simulink model "final_sim"  (R2024b)
settings: Solver=FixedStepAuto  StartTime=0.0  StopTime=10  FixedStep=step_size  RelTol=1e-3
values from neighbouring files (symbols this model uses):
  F_alphas = zeros([4,8])    [make_polynomial.m]
  Ic = I    (= 0)    [quadcopter_tmp_par.m]
  m = 4    [inertia.m]    (also in quadcopter_tmp_par.m)
  M_RB = [ m*eye(3) , zeros(3) ; zeros(3) , Ic2 ]    [inertia.m]    (also in quadcopter_tmp_par.m = [m*eye(3),zeros(3);zeros(3),Ic])
libraries: vrlib x3, aerolibutil x2, sharedtransform x2, simulink_extras x1, sharedutil x1
settings Model: Creator=vince  LastModifiedBy=vince

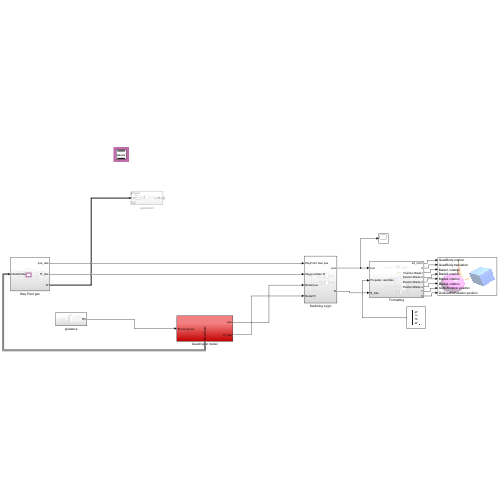
[thumbnail: Simulink's stored preview of the top-level diagram]
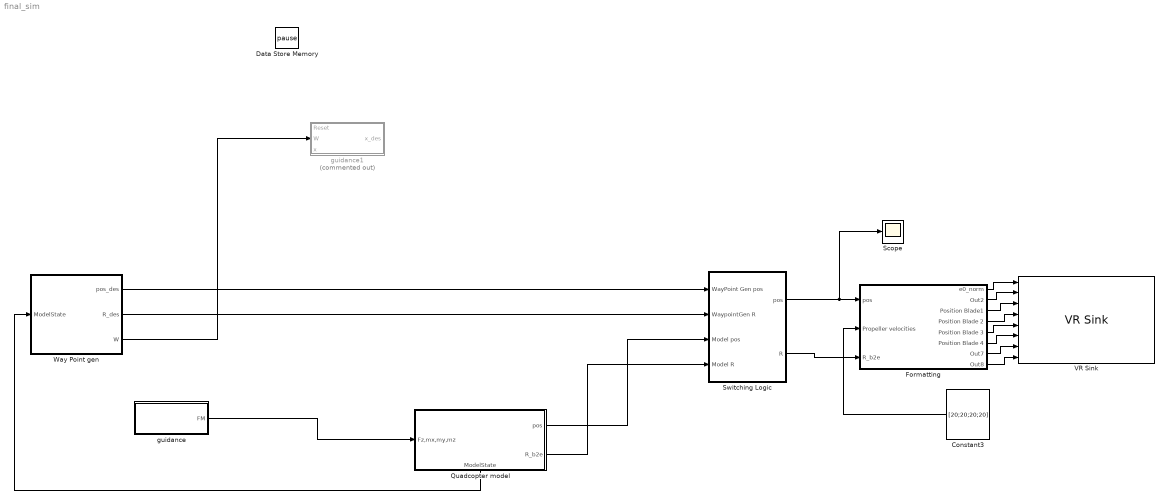
== system final_sim ==
  Constant3 : Constant  Value=[20;20;20;20]  VectorParams1D=off
  Data Store Memory : DataStoreMemory  DataStoreName=pause  WriteAfterWriteMsg=warning  ShowAdditionalParam=off  OutDataTypeStr=boolean
  Formatting : Subsystem
  Quadcopter model : Subsystem
      settings: PortSchema="{\"entries\":[{\"content\":{\"sides\":[{\"content\":{\"connectorIds\":[\"In1\"]},\"type\":\"ConnectorPlacement.EquallySpacedRectSide\",\"uuid\":\"b95d4d67-ceb1-468a-a740-70bed9055261\"},{\"content\":{\"connectorIds\":[\"Out1\",\"Out2\"],\"side\":\"RIGHT\"},\"type\":\"ConnectorPlacement.EquallySpacedRectSide\",\"uuid\":\"d9e2e888-327b-4c74-9853-42e66e59dabe\"},{\"content\":{\"side\":\"TOP\"},\"type\":\"ConnectorPlacement.EquallySpacedRectSide\",\"uuid\":\"f1e6c0a4-a009-4e38-aaef-f99bc46a780f\"},{\"content\":{\"connectorIds\":[\"Out3\"],\"side\":\"BOTTOM\"},\"type\":\"ConnectorPlacement.EquallySpacedRectSide\",\"uuid\":\"26785e0d-8be3-430d-abc1-8d415326c7f3\"}]},\"type\":\"ConnectorPlacement.EquallySpacedConnector\",\"uuid\":\"bfffa9f4-9135-40ac-b83a-608bfe18c3a4\"}],\"packageUris\":[\"http://schema.mathworks.com/mf0/Connector/R2020b\"],\"version\":\"1.0\"}"
  Scope : Scope
  Switching Logic : Subsystem
  VR Sink : vrlib/VR Sink  InstantiateOnLoad=on  SampleTime=12*0.005  ViewEnable=on  RemoteChange=off  RemoteView=off  FieldsWritten=QuadBody.rotation.4.1.1.double#QuadBody.translation.3.1.1.double#Blade1.rotation.4.1.1.double#Blade3.rotation.4.1.1.double#Blade2.rotation.4.1.1.double#Blade4.rotation.4.1.1.double#IsoNoRotation.position.3.1.1.double#OnQuadNoRotation.position.3.1.1.double  WorldFileName=Quadcopter_VR.wrl  AutoView=on  VideoDimensions=[]  AllowVariableSize=off  FigureProperties="{'Position', 'Name', 'Viewpoint', 'CameraBound', 'CameraDirection', 'CameraPosition', 'CameraUpVector', 'ZoomFactor', 'Antialiasing', 'Headlight', 'Lighting', 'Sound', 'StatusBar', 'Stereo3D', 'Stereo3DCameraOffset', 'Stereo3DHIT', 'ToolBar', 'Textures', 'Transparency', 'Triad', 'Wireframe', 'NavZones', 'NavMode', 'NavSpeed', 'CaptureFileFormat', 'CaptureFileName', 'Record2DCompressMethod', 'Record2DCompressQuality', 'Record2D', 'Record2DFileName', 'Record2DFPS', 'NavPanel'; [1.9301428571428571e+03   6.0471428571428555e+02   5.7600000000000000e+02   3.5000000000000000e+02], '', 'Chase - No Rotation', 'on', [0.0000000000000000e+00   0.0000000000000000e+00  -1.0000000000000000e+00], [0.0000000000000000e+00   0.0000000000000000e+00   0.0000000000000000e+00], [0.0000000000000000e+00   1.0000000000000000e+00   0.0000000000000000e+00], [1.0000000000000000e+00], 'on', 'on', 'on', 'on', 'on', 'off', [1.0000000149011612e-01], [0.0000000000000000e+00], 'on', 'on', 'on', 'none', 'off', 'off', 'fly', 'normal', 'tif', '%f_anim_%n.tif', 'auto', [7.5000000000000000e+01], 'off', '%f_anim_%n.avi', 'auto', 'halfbar'}"
  Way Point gen : Subsystem
  guidance : Subsystem
  guidance1 : Subsystem  Commented=on
  wires:
  Formatting/6(Position Blade 4) -> VR Sink/6
  Formatting/8(Out8) -> VR Sink/8
  Formatting/1(e0_norm) -> VR Sink/1
  Switching Logic/2(R) -> Formatting/3(R_b2e)
  Formatting/4(Position Blade 2) -> VR Sink/4
  Formatting/3(Position Blade1) -> VR Sink/3
  Formatting/7(Out7) -> VR Sink/7
  Formatting/5(Position Blade 3) -> VR Sink/5
  guidance/1(FM) -> Quadcopter model/1(Fz,mx,my,mz)
  Formatting/2(Out2) -> VR Sink/2
  Constant3/1 -> Formatting/2(Propeller velocities)
  Switching Logic/1(pos) -> Scope/1, Formatting/1(pos)
  Way Point gen/2(R_des) -> Switching Logic/2(WaypointGen R)
  Way Point gen/3(W) -> guidance1/2(W)
  Quadcopter model/2(R_b2e) -> Switching Logic/4(Model R)
  Way Point gen/1(pos_des) -> Switching Logic/1(WayPoint Gen pos)
  Quadcopter model/1(pos) -> Switching Logic/3(Model pos)
  Quadcopter model/3(ModelState) -> Way Point gen/1(ModelState)

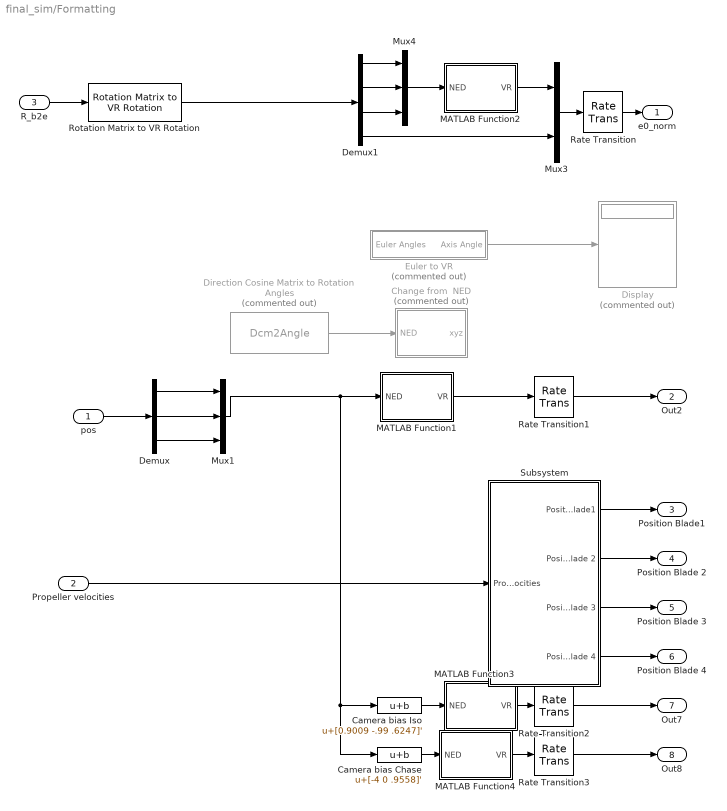
== system final_sim/Formatting ==
  pos : Inport
  Propeller velocities : Inport  Port=2
  R_b2e : Inport  Port=3
  Camera bias Chase : Bias  Bias=[-4 0 .9558]'  SaturateOnIntegerOverflow=off
  Camera bias Iso : Bias  Bias=[0.9009 -.99 .6247]'  SaturateOnIntegerOverflow=off
  Change from  NED : MATLAB Function  Commented=on  TreatAsAtomicUnit=on
  Demux : Demux  Outputs=3
  Demux1 : Demux
  Direction Cosine Matrix to Rotation Angles : Dcm2Angle  Commented=on
      settings: AttributesFormatString=Rotation Order: %<rotationOrder>
  Display : Display  Commented=on
  Euler to VR : Subsystem  Commented=on
  MATLAB Function1 : MATLAB Function  TreatAsAtomicUnit=on
  MATLAB Function2 : MATLAB Function  TreatAsAtomicUnit=on
  MATLAB Function3 : MATLAB Function  TreatAsAtomicUnit=on
  MATLAB Function4 : MATLAB Function  TreatAsAtomicUnit=on
  Mux1 : Mux  Inputs=3
  Mux3 : Mux  Inputs=2
  Mux4 : Mux  Inputs=3
  Rate Transition{,1..3} (4 alike) : RateTransition
  Rotation Matrix to VR Rotation : vrlib/Utilities/Rotation Matrix to VR Rotation  maxzero=1e-12
  Subsystem : Subsystem
  e0_norm : Outport
  Out2 : Outport  Port=2
  Position Blade1 : Outport  Port=3
  Position Blade 2 : Outport  Port=4
  Position Blade 3 : Outport  Port=5
  Position Blade 4 : Outport  Port=6
  Out7 : Outport  Port=7
  Out8 : Outport  Port=8
  wires:
  Rate Transition2/1 -> Out7/1
  Propeller velocities/1 -> Subsystem/1(Propeller velocities)
  Subsystem/3(Position Blade 3) -> Position Blade 3/1
  Subsystem/1(Position Blade1) -> Position Blade1/1
  Camera bias Chase/1 -> MATLAB Function4/1(NED)
  MATLAB Function4/1(VR) -> Rate Transition3/1
  Subsystem/2(Position Blade 2) -> Position Blade 2/1
  MATLAB Function3/1(VR) -> Rate Transition2/1
  MATLAB Function1/1(VR) -> Rate Transition1/1
  Rate Transition1/1 -> Out2/1
  Camera bias Iso/1 -> MATLAB Function3/1(NED)
  Mux1/1 -> MATLAB Function1/1(NED), Camera bias Chase/1, Camera bias Iso/1
  Rate Transition3/1 -> Out8/1
  Subsystem/4(Position Blade 4) -> Position Blade 4/1
  Demux/2 -> Mux1/2
  Demux/3 -> Mux1/3
  Demux/1 -> Mux1/1
  Euler to VR/1(Axis Angle) -> Display/1
  Direction Cosine Matrix to Rotation Angles/1 -> Change from  NED/1(NED)
  Demux1/1 -> Mux4/1
  Demux1/2 -> Mux4/2
  MATLAB Function2/1(VR) -> Mux3/1
  Mux4/1 -> MATLAB Function2/1(NED)
  Rotation Matrix to VR Rotation/1 -> Demux1/1
  Demux1/3 -> Mux4/3
  Mux3/1 -> Rate Transition/1
  Rate Transition/1 -> e0_norm/1
  Demux1/4 -> Mux3/2
  R_b2e/1 -> Rotation Matrix to VR Rotation/1
  pos/1 -> Demux/1

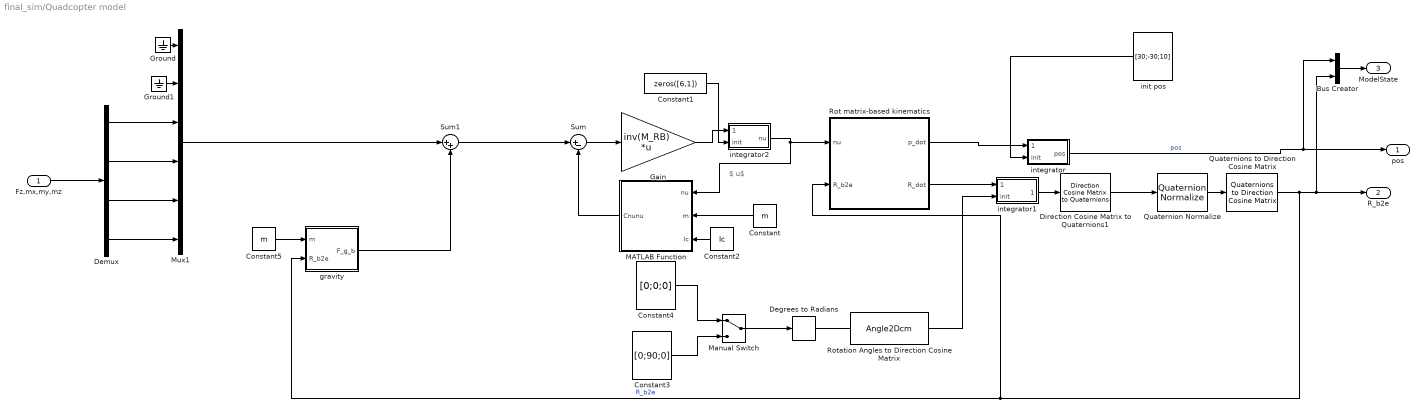
== system final_sim/Quadcopter model ==
  note: $\nu$
  Fz,mx,my,mz : Inport
  Bus Creator : BusCreator  Inputs=2  OutDataTypeStr=Bus: ModelStateBus
  Constant : Constant  Value=m
  Constant1 : Constant  Value=zeros([6,1])
  Constant2 : Constant  Value=Ic  VectorParams1D=off
  Constant3 : Constant  Value=[0;90;0]  VectorParams1D=off
  Constant4 : Constant  Value=[0;0;0]  VectorParams1D=off
  Constant5 : Constant  Value=m
  Degrees to Radians : simulink_extras/Transformations/Degrees to Radians
  Demux : Demux
  Direction Cosine Matrix to Quaternions1 : sharedtransform/Direction Cosine Matrix  to Quaternions  aMode=0  action=None  tolerance=eps(2)
  Gain : Gain  Gain=inv(M_RB)  Multiplication=Matrix(K*u) (u vector)
  Ground : Ground
  Ground1 : Ground
  MATLAB Function : MATLAB Function  TreatAsAtomicUnit=on
  Manual Switch : ManualSwitch
  Mux1 : Mux  Inputs=6
  Quaternion Normalize : sharedutil/Quaternion Normalize  aMode=aMode
  Quaternions to Direction Cosine Matrix : sharedtransform/Quaternions to  Direction Cosine Matrix  aMode=aMode
  Rot matrix-based kinematics : Subsystem
  Rotation Angles to Direction Cosine Matrix : Angle2Dcm
      settings: AttributesFormatString=Rotation Order: %<rotationOrder>
  Sum : Sum  Inputs=|+-
  Sum1 : Sum  Inputs=|++
  gravity : MATLAB Function  TreatAsAtomicUnit=on
  init pos : Constant  Value=[30;-30;10]  VectorParams1D=off
  integrator : Subsystem
  integrator1 : Subsystem
  integrator2 : Subsystem
  pos : Outport
  R_b2e : Outport  Port=2
  ModelState : Outport  Port=3
  wires:
  Constant/1 -> MATLAB Function/2(m)
  Degrees to Radians/1 -> ?
  Constant2/1 -> MATLAB Function/3(Ic)
  Constant4/1 -> Manual Switch/1
  MATLAB Function/1(Cnunu) -> Sum/2
  Gain/1 -> integrator2/1(nu_dot)
  Constant3/1 -> Manual Switch/2
  Rotation Angles to Direction Cosine Matrix/1 -> integrator1/2(init)
  Sum/1 -> Gain/1
  Manual Switch/1 -> Degrees to Radians/1
  Rot matrix-based kinematics/1(p_dot) -> integrator/1(p_dot)
  Rot matrix-based kinematics/2(R_dot) -> integrator1/1(R_odtt)
  integrator/1(pos) -> Bus Creator/1, pos/1  "pos"
  Demux/4 -> Mux1/6
  Demux/3 -> Mux1/5
  Demux/2 -> Mux1/4
  Fz,mx,my,mz/1 -> Demux/1
  Ground/1 -> Mux1/1
  Ground1/1 -> Mux1/2
  Quaternion Normalize/1 -> Quaternions to Direction Cosine Matrix/1
  Constant5/1 -> gravity/1(m)
  gravity/1(F_g_b) -> Sum1/2
  Sum1/1 -> Sum/1
  Demux/1 -> Mux1/3
  integrator2/1(nu) -> MATLAB Function/1(nu), Rot matrix-based kinematics/1(nu)
  Direction Cosine Matrix to Quaternions1/1 -> Quaternion Normalize/1
  integrator1/1(R_b2e) -> Direction Cosine Matrix to Quaternions1/1
  Mux1/1 -> Sum1/1
  Quaternions to Direction Cosine Matrix/1 -> Bus Creator/2, R_b2e/1, Rot matrix-based kinematics/2(R_b2e), gravity/2(R_b2e)  "R_b2e"
  init pos/1 -> integrator/2(init)
  Constant1/1 -> integrator2/2(init)
  Bus Creator/1 -> ModelState/1

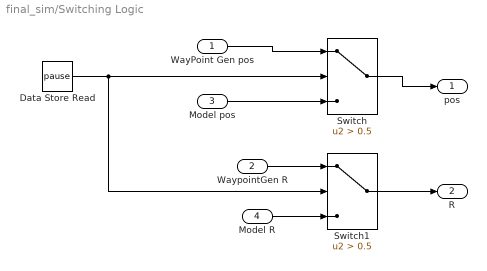
== system final_sim/Switching Logic ==
  WayPoint Gen pos : Inport
  WaypointGen R : Inport  Port=2
  Model pos : Inport  Port=3
  Model R : Inport  Port=4
  Data Store Read : DataStoreRead  DataStoreName=pause  IndexOptions=Index vector (dialog)  Indices=1  OutputSizes=1
  Switch : Switch  Criteria=u2 > Threshold  Threshold=0.5  SaturateOnIntegerOverflow=off  InputSameDT=off
  Switch1 : Switch  Criteria=u2 > Threshold  Threshold=0.5  SaturateOnIntegerOverflow=off  InputSameDT=off
  pos : Outport
  R : Outport  Port=2
  wires:
  Model pos/1 -> Switch/3
  Data Store Read/1 -> Switch1/2, Switch/2
  WayPoint Gen pos/1 -> Switch/1
  Switch/1 -> pos/1
  WaypointGen R/1 -> Switch1/1
  Model R/1 -> Switch1/3
  Switch1/1 -> R/1

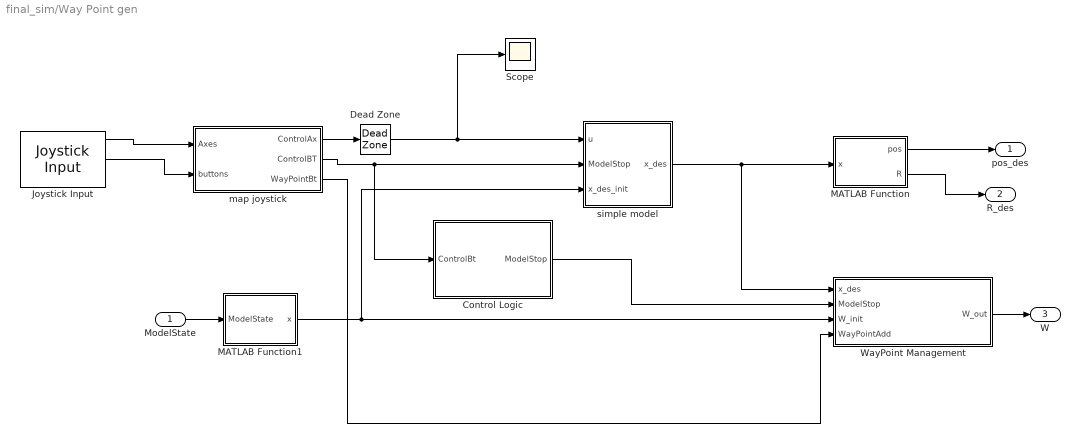
== system final_sim/Way Point gen ==
  ModelState : Inport
  Control Logic : Subsystem
  Dead Zone : DeadZone  LowerValue=-0.1  UpperValue=0.1
  Joystick Input : vrlib/Joystick Input  joyid=1  adjustports=on  forcefeed=off
  MATLAB Function : MATLAB Function  TreatAsAtomicUnit=on
  MATLAB Function1 : MATLAB Function  TreatAsAtomicUnit=on
  Scope : Scope
  WayPoint Management : MATLAB Function  TreatAsAtomicUnit=on
  map joystick : MATLAB Function  TreatAsAtomicUnit=on
  simple model : Subsystem
  pos_des : Outport
  R_des : Outport  Port=2
  W : Outport  Port=3
  wires:
  Joystick Input/2 -> map joystick/2(buttons)
  Joystick Input/1 -> map joystick/1(Axes)
  map joystick/1(ControlAx) -> Dead Zone/1
  Dead Zone/1 -> Scope/1, simple model/1(u)
  map joystick/2(ControlBT) -> Control Logic/1(ControlBt), simple model/2(ModelStop)
  simple model/1(x_des) -> MATLAB Function/1(x), WayPoint Management/1(x_des)
  map joystick/3(WayPointBt) -> WayPoint Management/4(WayPointAdd)
  WayPoint Management/1(W_out) -> W/1
  MATLAB Function/1(pos) -> pos_des/1
  MATLAB Function/2(R) -> R_des/1
  MATLAB Function1/1(x) -> WayPoint Management/3(W_init), simple model/3(x_des_init)
  ModelState/1 -> MATLAB Function1/1(ModelState)
  Control Logic/1(ModelStop) -> WayPoint Management/2(ModelStop)

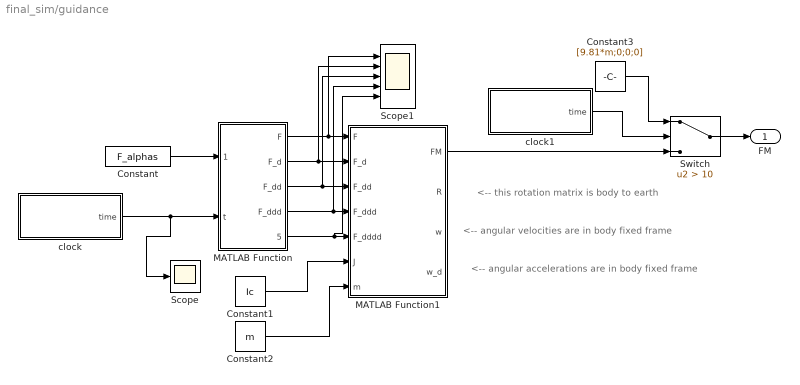
== system final_sim/guidance ==
  note: <-- angular velocities are in body fixed frame
  note: <-- this rotation matrix is body to earth
  note: <-- angular accelerations are in body fixed frame
  Constant : Constant  Value=F_alphas
  Constant1 : Constant  Value=Ic
  Constant2 : Constant  Value=m
  Constant3 : Constant  Value=[9.81*m;0;0;0]
  MATLAB Function : MATLAB Function  TreatAsAtomicUnit=on
  MATLAB Function1 : MATLAB Function  TreatAsAtomicUnit=on
  Scope : Scope
  Scope1 : Scope  NumInputPorts=5
  Switch : Switch  Criteria=u2 > Threshold  Threshold=10  SaturateOnIntegerOverflow=off  InputSameDT=off
  clock : Subsystem
  clock1 : Subsystem
  FM : Outport
  wires:
  Constant/1 -> MATLAB Function/1(F_alphas)
  MATLAB Function/1(F) -> Scope1/1, MATLAB Function1/1(F)
  MATLAB Function/2(F_d) -> Scope1/2, MATLAB Function1/2(F_d)
  MATLAB Function/3(F_dd) -> Scope1/3, MATLAB Function1/3(F_dd)
  MATLAB Function/4(F_ddd) -> Scope1/4, MATLAB Function1/4(F_ddd)
  MATLAB Function/5(F_dddd) -> Scope1/5, MATLAB Function1/5(F_dddd)
  Constant1/1 -> MATLAB Function1/6(J)
  Constant2/1 -> MATLAB Function1/7(m)
  MATLAB Function1/1(FM) -> Switch/3
  Switch/1 -> FM/1
  clock1/1(time) -> Switch/2
  Constant3/1 -> Switch/1
  clock/1(time) -> Scope/1, MATLAB Function/2(t)

== system final_sim/guidance1 ==
  Reset : Inport
  W : Inport  Port=2
  x : Inport  Port=3
  select way point : MATLAB Function  TreatAsAtomicUnit=on
  x_des : Outport
  wires:
  W/1 -> select way point/1(W)
  x/1 -> select way point/2(x)
  select way point/1(x_des) -> x_des/1
  Reset/1 -> select way point/3(reset)

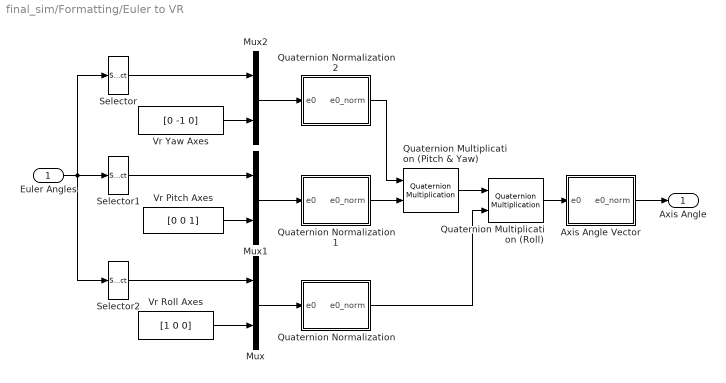
== system final_sim/Formatting/Euler to VR ==
  Euler Angles : Inport
  Axis Angle Vector : Subsystem
  Mux : Mux  Inputs=2
  Mux1 : Mux  Inputs=2
  Mux2 : Mux  Inputs=2
  Quaternion Multiplication (Pitch & Yaw) : aerolibutil/Quaternion Multiplication
  Quaternion Multiplication (Roll) : aerolibutil/Quaternion Multiplication
  Quaternion Normalization : Subsystem
  Quaternion Normalization1 : Subsystem
  Quaternion Normalization2 : Subsystem
  Selector : Selector  InputPortWidth=3  IndexOptions=Index vector (dialog)  Indices=[3]  OutputSizes=1
  Selector1 : Selector  InputPortWidth=3  IndexOptions=Index vector (dialog)  Indices=[2]  OutputSizes=1
  Selector2 : Selector  InputPortWidth=3  IndexOptions=Index vector (dialog)  Indices=[1]  OutputSizes=1
  Vr Pitch Axes : Constant  Value=[0 0 1]
  Vr Roll Axes : Constant  Value=[1 0 0]
  Vr Yaw Axes : Constant  Value=[0 -1 0]
  Axis Angle : Outport  VectorParamsAs1DForOutWhenUnconnected=off
  wires:
  Quaternion Multiplication (Roll)/1 -> Axis Angle Vector/1(e0)
  Axis Angle Vector/1(e0_norm) -> Axis Angle/1
  Quaternion Normalization/1(e0_norm) -> Quaternion Multiplication (Roll)/2
  Quaternion Normalization2/1(e0_norm) -> Quaternion Multiplication (Pitch & Yaw)/1
  Quaternion Normalization1/1(e0_norm) -> Quaternion Multiplication (Pitch & Yaw)/2
  Mux2/1 -> Quaternion Normalization2/1(e0)
  Mux1/1 -> Quaternion Normalization1/1(e0)
  Mux/1 -> Quaternion Normalization/1(e0)
  Selector/1 -> Mux2/1
  Vr Yaw Axes/1 -> Mux2/2
  Selector1/1 -> Mux1/1
  Vr Pitch Axes/1 -> Mux1/2
  Selector2/1 -> Mux/1
  Vr Roll Axes/1 -> Mux/2
  Euler Angles/1 -> Selector2/1, Selector1/1, Selector/1
  Quaternion Multiplication (Pitch & Yaw)/1 -> Quaternion Multiplication (Roll)/1

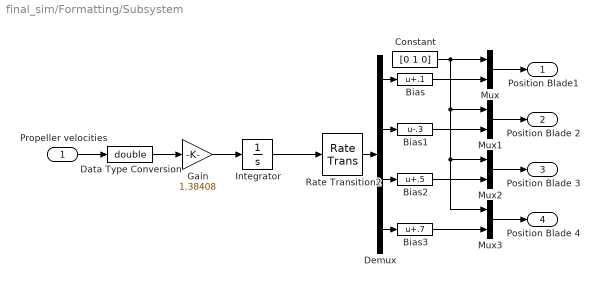
== system final_sim/Formatting/Subsystem ==
  Propeller velocities : Inport
  Bias : Bias  Bias=.1  SaturateOnIntegerOverflow=off
  Bias1 : Bias  Bias=-.3  SaturateOnIntegerOverflow=off
  Bias2 : Bias  Bias=.5  SaturateOnIntegerOverflow=off
  Bias3 : Bias  Bias=.7  SaturateOnIntegerOverflow=off
  Constant : Constant  Value=[0 1 0]
  Data Type Conversion : DataTypeConversion  OutDataTypeStr=double  SaturateOnIntegerOverflow=off  RndMeth=Floor
  Demux : Demux
  Gain : Gain  Gain=1.38408
  Integrator : Integrator  InitialCondition=[.1 ; .2 ;-.3 ;-.4]  WrapState=on  WrappedStateUpperValue=2*pi  WrappedStateLowerValue=-2*pi
  Mux{,1..3} (4 alike) : Mux  Inputs=2
  Rate Transition2 : RateTransition
  Position Blade1 : Outport  VectorParamsAs1DForOutWhenUnconnected=off
  Position Blade 2 : Outport  Port=2  VectorParamsAs1DForOutWhenUnconnected=off
  Position Blade 3 : Outport  Port=3  VectorParamsAs1DForOutWhenUnconnected=off
  Position Blade 4 : Outport  Port=4  VectorParamsAs1DForOutWhenUnconnected=off
  wires:
  Bias3/1 -> Mux3/2
  Mux3/1 -> Position Blade 4/1
  Bias1/1 -> Mux1/2
  Bias2/1 -> Mux2/2
  Demux/2 -> Bias1/1
  Constant/1 -> Mux3/1, Mux2/1, Mux1/1, Mux/1
  Mux1/1 -> Position Blade 2/1
  Mux2/1 -> Position Blade 3/1
  Integrator/1 -> Rate Transition2/1
  Mux/1 -> Position Blade1/1
  Demux/3 -> Bias2/1
  Bias/1 -> Mux/2
  Propeller velocities/1 -> Data Type Conversion/1
  Demux/4 -> Bias3/1
  Rate Transition2/1 -> Demux/1
  Demux/1 -> Bias/1
  Data Type Conversion/1 -> Gain/1
  Gain/1 -> Integrator/1

== system final_sim/Quadcopter model/Rot matrix-based kinematics ==
  nu : Inport
  R_b2e : Inport  Port=2
  MATLAB Function : MATLAB Function  TreatAsAtomicUnit=on
  p_dot : Outport
  R_dot : Outport  Port=2
  wires:
  MATLAB Function/2(R_dot) -> R_dot/1
  nu/1 -> MATLAB Function/1(nu)
  R_b2e/1 -> MATLAB Function/2(R_b2e)
  MATLAB Function/1(p_dot) -> p_dot/1

== system final_sim/Quadcopter model/integrator ==
  p_dot : Inport
  init : Inport  Port=2
  Constant : Constant  Value=0
  Data Store Read : DataStoreRead  DataStoreName=pause  IndexOptions=Index vector (dialog)  Indices=1  OutputSizes=1
  Integrator : Integrator  InitialConditionSource=external
  Switch : Switch  Criteria=u2 > Threshold  SaturateOnIntegerOverflow=off  InputSameDT=off
  pos : Outport
  wires:
  Data Store Read/1 -> Switch/2
  p_dot/1 -> Switch/3
  Integrator/1 -> pos/1
  init/1 -> Integrator/2
  Constant/1 -> Switch/1
  Switch/1 -> Integrator/1

== system final_sim/Quadcopter model/integrator1 ==
  R_odtt : Inport
  init : Inport  Port=2
  Constant : Constant  Value=0
  Data Store Read : DataStoreRead  DataStoreName=pause  IndexOptions=Index vector (dialog)  Indices=1  OutputSizes=1
  Integrator : Integrator  InitialConditionSource=external
  Switch : Switch  Criteria=u2 > Threshold  SaturateOnIntegerOverflow=off  InputSameDT=off
  R_b2e : Outport
  wires:
  Data Store Read/1 -> Switch/2
  R_odtt/1 -> Switch/3
  Integrator/1 -> R_b2e/1
  init/1 -> Integrator/2
  Constant/1 -> Switch/1
  Switch/1 -> Integrator/1

== system final_sim/Quadcopter model/integrator2 ==
  nu_dot : Inport
  init : Inport  Port=2
  Constant : Constant  Value=0
  Data Store Read : DataStoreRead  DataStoreName=pause  IndexOptions=Index vector (dialog)  Indices=1  OutputSizes=1
  Integrator : Integrator  InitialConditionSource=external
  Switch : Switch  Criteria=u2 > Threshold  SaturateOnIntegerOverflow=off  InputSameDT=off
  nu : Outport
  wires:
  Data Store Read/1 -> Switch/2
  nu_dot/1 -> Switch/3
  Integrator/1 -> nu/1
  init/1 -> Integrator/2
  Constant/1 -> Switch/1
  Switch/1 -> Integrator/1

== system final_sim/Way Point gen/Control Logic ==
  ControlBt : Inport
  Control Logic : MATLAB Function  Priority=0  TreatAsAtomicUnit=on
  ModelStop : Outport
  wires:
  ControlBt/1 -> Control Logic/1(ControlBt)
  Control Logic/1(ModelStop) -> ModelStop/1

== system final_sim/Way Point gen/simple model ==
  u : Inport
  ModelStop : Inport  Port=2
  x_des_init : Inport  Port=3
  Gain : Gain
  Integrator : Integrator  ExternalReset=rising  InitialConditionSource=external
  x_des : Outport
  wires:
  Gain/1 -> Integrator/1
  x_des_init/1 -> Integrator/3
  u/1 -> Gain/1
  ModelStop/1 -> Integrator/2
  Integrator/1 -> x_des/1

== system final_sim/guidance/clock ==
  Clock : Clock
  Data Store Read : DataStoreRead  DataStoreName=pause  IndexOptions=Index vector (dialog)  Indices=1  OutputSizes=1
  MATLAB Function : MATLAB Function  TreatAsAtomicUnit=on
  time : Outport
  wires:
  Clock/1 -> MATLAB Function/1(time)
  Data Store Read/1 -> MATLAB Function/2(pause)
  MATLAB Function/1(time_out) -> time/1

== system final_sim/guidance/clock1 ==
  Clock : Clock
  Data Store Read : DataStoreRead  DataStoreName=pause  IndexOptions=Index vector (dialog)  Indices=1  OutputSizes=1
  MATLAB Function : MATLAB Function  TreatAsAtomicUnit=on
  time : Outport
  wires:
  Clock/1 -> MATLAB Function/1(time)
  Data Store Read/1 -> MATLAB Function/2(pause)
  MATLAB Function/1(time_out) -> time/1

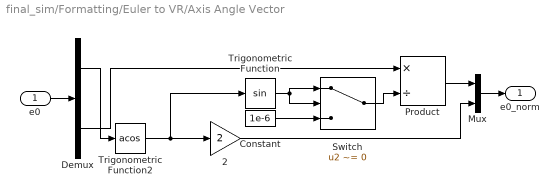
== system final_sim/Formatting/Euler to VR/Axis Angle Vector ==
  e0 : Inport
  2 : Gain  Gain=2  SaturateOnIntegerOverflow=on  OutDataTypeStr=Inherit: Same as input  ParamDataTypeStr=Inherit: Same as input
  Constant : Constant  Value=1e-6
  Demux : Demux  Outputs=[1 3 ]
      settings: DisplayOption=none
  Mux : Mux  Inputs=2
  Product : Product  Inputs=*/  InputSameDT=on  SaturateOnIntegerOverflow=on  OutDataTypeStr=Inherit: Same as first input
  Switch : Switch  Criteria=u2 ~= 0  SaturateOnIntegerOverflow=off  InputSameDT=off
  Trigonometric Function : Trigonometry
  Trigonometric Function2 : Trigonometry  Operator=acos
  e0_norm : Outport  VectorParamsAs1DForOutWhenUnconnected=off
  wires:
  Demux/1 -> Trigonometric Function2/1
  Demux/2 -> Product/1
  Mux/1 -> e0_norm/1
  Product/1 -> Mux/1
  2/1 -> Mux/2
  Trigonometric Function/1 -> Switch/1, Switch/2
  Trigonometric Function2/1 -> Trigonometric Function/1, 2/1
  e0/1 -> Demux/1
  Constant/1 -> Switch/3
  Switch/1 -> Product/2

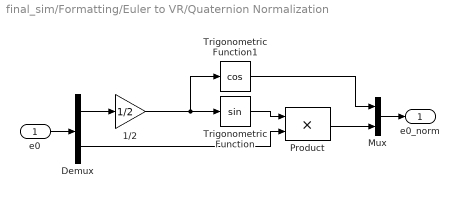
== system final_sim/Formatting/Euler to VR/Quaternion Normalization ==
  e0 : Inport
  1/2 : Gain  Gain=1/2  SaturateOnIntegerOverflow=on  OutDataTypeStr=Inherit: Same as input  ParamDataTypeStr=Inherit: Same as input
  Demux : Demux  Outputs=[1 3]
      settings: DisplayOption=none
  Mux : Mux  Inputs=2
  Product : Product  InputSameDT=on  SaturateOnIntegerOverflow=on  OutDataTypeStr=Inherit: Same as first input
  Trigonometric Function : Trigonometry
  Trigonometric Function1 : Trigonometry  Operator=cos
  e0_norm : Outport  VectorParamsAs1DForOutWhenUnconnected=off
  wires:
  Trigonometric Function1/1 -> Mux/1
  Demux/2 -> Product/2
  Demux/1 -> 1/2/1
  Mux/1 -> e0_norm/1
  Product/1 -> Mux/2
  Trigonometric Function/1 -> Product/1
  1/2/1 -> Trigonometric Function1/1, Trigonometric Function/1
  e0/1 -> Demux/1

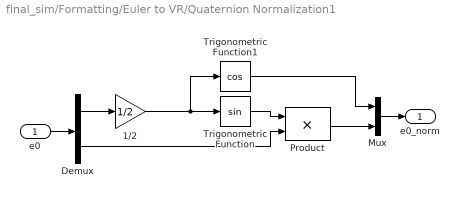
== system final_sim/Formatting/Euler to VR/Quaternion Normalization1 ==
  e0 : Inport
  1/2 : Gain  Gain=1/2  SaturateOnIntegerOverflow=on  OutDataTypeStr=Inherit: Same as input  ParamDataTypeStr=Inherit: Same as input
  Demux : Demux  Outputs=[1 3]
      settings: DisplayOption=none
  Mux : Mux  Inputs=2
  Product : Product  InputSameDT=on  SaturateOnIntegerOverflow=on  OutDataTypeStr=Inherit: Same as first input
  Trigonometric Function : Trigonometry
  Trigonometric Function1 : Trigonometry  Operator=cos
  e0_norm : Outport  VectorParamsAs1DForOutWhenUnconnected=off
  wires:
  e0/1 -> Demux/1
  1/2/1 -> Trigonometric Function/1, Trigonometric Function1/1
  Trigonometric Function/1 -> Product/1
  Product/1 -> Mux/2
  Mux/1 -> e0_norm/1
  Demux/1 -> 1/2/1
  Demux/2 -> Product/2
  Trigonometric Function1/1 -> Mux/1

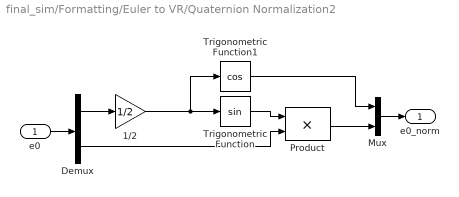
== system final_sim/Formatting/Euler to VR/Quaternion Normalization2 ==
  e0 : Inport
  1/2 : Gain  Gain=1/2  SaturateOnIntegerOverflow=on  OutDataTypeStr=Inherit: Same as input  ParamDataTypeStr=Inherit: Same as input
  Demux : Demux  Outputs=[1 3]
      settings: DisplayOption=none
  Mux : Mux  Inputs=2
  Product : Product  InputSameDT=on  SaturateOnIntegerOverflow=on  OutDataTypeStr=Inherit: Same as first input
  Trigonometric Function : Trigonometry
  Trigonometric Function1 : Trigonometry  Operator=cos
  e0_norm : Outport  VectorParamsAs1DForOutWhenUnconnected=off
  wires:
  Trigonometric Function1/1 -> Mux/1
  Demux/2 -> Product/2
  Demux/1 -> 1/2/1
  Mux/1 -> e0_norm/1
  Product/1 -> Mux/2
  Trigonometric Function/1 -> Product/1
  1/2/1 -> Trigonometric Function1/1, Trigonometric Function/1
  e0/1 -> Demux/1

== matlab function final_sim/guidance/MATLAB Function1 ==
  data: F input; FM output; F_d input; F_dd input; F_ddd input; F_dddd input; J input; m input; R output; w output; w_d output
function [FM,R,w,w_d]  = fcn(F,F_d,F_dd,F_ddd,F_dddd,J,m)

g=9.81;


%physical quantities and vectors
a=F_dd(1:3); %acceleration
j=F_ddd(1:3); %jerk
s=F_dddd(1:3); %snap


%rotation matrix constants
psi=F(4);
x_c=[ cos(psi);  sin(psi);   0];
y_c=[-sin(psi);  cos(psi);    0];
alpha=a+g*[0;0;1];


%rotation matrix vectors
x_b=cross(y_c,alpha);
x_b=x_b/norm(x_b);
y_b=cross(alpha,x_b);
y_b=y_b/norm(y_b);
z_b=cross(x_b,y_b);
R=[x_b,y_b,z_b];


%Thrust
c=z_b'*alpha;
T=m*c;

%constants
B1=c;
D1=x_b'*j;
A2=c;
D2=-y_b'*j;
B3=-y_c'*z_b;
C3=norm(cross(y_c,z_b));
D3=F_d(4)*x_c'*x_b;


%angluar velocities
w_x=D2/A2;
w_y=D1/B1;
w_z=(B1*D3-B3*D1)/(B1*C3);
w=[w_x;w_y;w_z];


%more physical quantities
c_dot=z_b'*j;

%more constants
e1=x_b'*s-2*c_dot*w_y-c*w_x*w_z;
e2=-y_b'*s-2*c_dot*w_x+c*w_y*w_z;
e3=F_dd(4)*x_c'*x_b+2*F_d(4)*w_z*x_c'*y_b-2*F_d(4)*w_y*x_c'*z_b-w_x*w_y*y_c'*y_b-w_x*w_z*y_c'*z_b;
% e31=F_dd(4)*x_c'*x_b;
% e32=-2*F_d(4)*w_z*x_c'*y_b;
% e33=+2*F_d(4)*w_y*x_c'*z_b;
% e34=-w_x*w_y*y_c'*y_b;
% e35=+w_x*w_z*y_c'*z_b;
% e=[e31;e32;e33;e34;e35];
% e3=e31+e32+e33+e34+e35;
% 
% 
w_d_x=(e2)/(A2);
w_d_y=(e1)/(B1);
w_d_z=(B1*e3-B3*e1)/(B1*C3);
w_d=[w_d_x;w_d_y;w_d_z];

% J_x=J(1,1);
% J_y=J(2,2);
% J_z=J(3,3);
% 
% % tau_x=J_x*w_d_x+(J_z-J_y)*w_y*w_z;
% % tau_y=J_y*w_d_y+(J_x-J_z)*w_x*w_z;
% % tau_z=J_z*w_d_z+(J_y-J_x)*w_y*w_x;
% 
M=J*w_d+cross(w,J*w);
% 
FM=[T;M];
% FM=[T;0;0;0];

== matlab function final_sim/guidance/clock/MATLAB Function ==
  settings: updateMethod=DISCRETE
  data: time input; time_out output; pause input
function time_out = fcn(time,pause)

persistent old_time;
persistent t_offset;

if isempty(t_offset)
    t_offset=0;
    old_time=0;
end

if pause==true
    t_offset=time-old_time;
else
    old_time=time;
end

time_out=time-t_offset;

== matlab function final_sim/Quadcopter model/Rot matrix-based kinematics/MATLAB Function ==
  data: nu input; p_dot output; R_b2e input; R_dot output
function [p_dot,R_dot] = fcn(nu,R_b2e)
v_b=nu(1:3);
w_b=nu(4:6);
p_dot=R_b2e*v_b;
omega_cross=[0,-w_b(3),w_b(2);
             w_b(3),0,-w_b(1);
             -w_b(2),w_b(1),0];
R_dot=R_b2e*omega_cross;

== matlab function final_sim/Formatting/MATLAB Function1 ==
  data: NED input; VR output
function VR = NED2VR(NED)

x = NED(1); % north
y = NED(2); % east 
z = NED(3); % down

VR = [ x ; z ; -y ];

== matlab function final_sim/Formatting/MATLAB Function3 ==
  data: NED input; VR output
function VR = NED2VR(NED)

x = NED(1); % north
y = NED(2); % east 
z = NED(3); % down

VR = [ x ; z ; -y ];

== matlab function final_sim/Formatting/MATLAB Function4 ==
  data: NED input; VR output
function VR = NED2VR(NED)

x = NED(1); % north
y = NED(2); % east 
z = NED(3); % down

VR = [ x ; z ; -y ];

== matlab function final_sim/Way Point gen/MATLAB Function1 ==
  data: ModelState input Bus: ModelStateBus; x output
function x = fcn(ModelState)

x=zeros([4,1]);
x(1:3)=ModelState.pos;
angles=rotm2eul(ModelState.R_b2e);
x(4)=angles(3);

== matlab function final_sim/guidance/clock1/MATLAB Function ==
  settings: updateMethod=DISCRETE
  data: time input; time_out output; pause input
function time_out = fcn(time,pause)

persistent old_time;
persistent t_offset;

if isempty(t_offset)
    t_offset=0;
    old_time=0;
end

if pause==true
    t_offset=time-old_time;
else
    old_time=time;
end

time_out=time-t_offset;

== matlab function final_sim/Formatting/Change from  NED ==
  data: NED input; xyz output
function xyz = fcn(NED)
xyz=zeros([4,1]);
xyz(1)=NED(1);
xyz(2)=-NED(3);
xyz(3)=NED(2);
xyz(4)=NED(4);

== matlab function final_sim/Quadcopter model/MATLAB Function ==
  data: nu input; Cnunu output; m input; Ic input
function Cnunu = fcn(nu,m,Ic)

v = nu(1:3);  % linear velocities (expressed in the body frame)
omega = nu(4:6); % angular velocities (expressed in the body frame)

% Coriolis term
Cnunu = [ cross(omega,m*v) ; -cross(Ic*omega,omega) ];

== matlab function final_sim/Way Point gen/WayPoint Management ==
  settings: updateMethod=DISCRETE  sampleTime=step_size
  data: x_des input; ModelStop input; W_init input; W_out output size=[4,inf]; WayPointAdd input
function W_out = fcn(x_des, ModelStop,W_init,WayPointAdd)

persistent W;
if isempty(W)
    W=zeros([4,0]);
end

persistent WPAdd_prev;
if isempty(WPAdd_prev)
    WPAdd_prev=WayPointAdd;
end

persistent ModStop_prev
if isempty(ModStop_prev)
    ModStop_prev=ModelStop;
end

if ModelStop==true & ModStop_prev==false
    W=zeros([4,0]);
end

if WayPointAdd==true & WPAdd_prev==false
    W=[W,x_des];
end

if size(W,2)==0
    W_out=W_init;
else
    W_out=W;
end

WPAdd_prev=WayPointAdd;
ModStop_prev=ModelStop;

== matlab function final_sim/Quadcopter model/gravity ==
  data: m input; R_b2e input; F_g_b output
function F_g_b = fcn(m,R_b2e)
F_g=[0;0;-m*9.81];
F_g_b=[R_b2e'*F_g;0;0;0];

== matlab function final_sim/Way Point gen/Control Logic/Control Logic ==
  settings: updateMethod=DISCRETE  sampleTime=0.01
  data: ControlBt input; ModelStop output; pause data_store_memory
function ModelStop   = fcn(ControlBt)

persistent CBT_prev;
global pause;
persistent ModStop;

%initialization
if isempty(CBT_prev)
    CBT_prev=ControlBt;

    %outputs
    ModStop=false;
    ModelStop=false;
    return
end

%state update
if ControlBt==true & CBT_prev==false 
    ModStop=~ModStop;
    pause=ModStop;
end

%outputs
ModelStop=ModStop;


%update internal
CBT_prev=ControlBt;

== matlab function final_sim/Way Point gen/MATLAB Function ==
  data: x input; pos output; R output
function [pos,R] = fcn(x)

pos=x(1:3);
yaw=x(4);

R=[cos(yaw),-sin(yaw),0;
    sin(yaw),cos(yaw),0;
    0,0,1];

== matlab function final_sim/Way Point gen/map joystick ==
  data: Axes input; ControlAx output; buttons input; ControlBT output; WayPointBt output
function [ControlAx,ControlBT,WayPointBt] = fcn(Axes,buttons)
%ax 3,1,2,4 bt 1,2
%ps4 2,3,6,1 bt 
ControlAx=Axes([6,3,2,1]).*[-1;1;1;1];
ControlBT=buttons(3);
WayPointBt=buttons(2);

== matlab function final_sim/Formatting/MATLAB Function2 ==
  data: NED input; VR output
function VR = NED2VR(NED)

x = NED(1); % north
y = NED(2); % east 
z = NED(3); % down

VR = [ x ; z ; -y ];

== matlab function final_sim/guidance1/select way point ==
  settings: updateMethod=DISCRETE
  data: W input size=[4,inf]; x_des output; x input size=[4,1]; reset input
function x_des = fcn(W,x,reset)

persistent i;
if isempty(i)
    i=1;
end

if reset==true
    i=1;
    x_des=zeros([4,1]);
    return;
end



thres=0.2;
if norm(W(:,i)-x)<=thres
    i=i+1;
    if i>size(W,2)
        i=size(W,2);
    end
end

x_des=zeros([4,1]);
x_des(:)=W(:,i);

== matlab function final_sim/guidance/MATLAB Function ==
  data: F_alphas input; F output; t input; F_d output; F_dd output; F_ddd output; F_dddd output
function [F,F_d,F_dd,F_ddd,F_dddd] = fcn(F_alphas,t)
b=      [1,   t,    t^2,    t^3,        t^4,        t^5,        t^6,        t^7];
b_p=    [0,   1,    2*t,  3*t^2,      4*t^3,      5*t^4,      6*t^5,      7*t^6];
b_pp=   [0,   0,      2,  3*2*t,    4*3*t^2,    5*4*t^3,    6*5*t^4,    7*6*t^5];
b_ppp=  [0,   0,      0,    3*2,    4*3*2*t,  5*4*3*t^2,  6*5*4*t^3,  7*6*5*t^4];
b_pppp= [0,   0,      0,      0,      4*3*2,  5*4*3*2*t,6*5*4*3*t^2,7*6*5*4*t^3];

% b=      [1,   t,    t^2,    t^3,        t^4,        t^5];
% b_p=    [0,   1,    2*t,  3*t^2,      4*t^3,      5*t^4];
% b_pp=   [0,   0,      2,  3*2*t,    4*3*t^2,    5*4*t^3];
% b_ppp=  [0,   0,      0,    3*2,    4*3*2*t,  5*4*3*t^2];
% b_pppp= [0,   0,      0,      0,      4*3*2,  5*4*3*2*t];


F=F_alphas*b';
F_d=F_alphas*b_p';
F_dd=F_alphas*b_pp';
F_ddd=F_alphas*b_ppp';
F_dddd=F_alphas*b_pppp';
